simulink model "ES200A_CurrMeas"  (R2013b)
settings: Solver=FixedStepDiscrete  SolverMode=SingleTasking  StartTime=0.0  StopTime=1  FixedStep=0.000125  RelTol=1e-3
values from neighbouring files (symbols this model uses):
  ARCHGLBPRM_2PI_ULS_F32 = DataDict.Constant    [ES200A_CurrMeas_DataDict.m]
  CurrMeasEolGainMax = DataDict.Calibration    [ES200A_CurrMeas_DataDict.m]
  CurrMeasEolGainMin = DataDict.Calibration    [ES200A_CurrMeas_DataDict.m]
  CurrMeasEolGainNrOfSample = DataDict.Calibration    [ES200A_CurrMeas_DataDict.m]
  CurrMeasEolGainNumer = DataDict.Calibration    [ES200A_CurrMeas_DataDict.m]
  CurrMeasEolMaxMotVel = DataDict.Calibration    [ES200A_CurrMeas_DataDict.m]
  CurrMeasEolOffsHiBrdgVltgMin = DataDict.Calibration    [ES200A_CurrMeas_DataDict.m]
  CurrMeasEolOffsHiCmuOffs = DataDict.Calibration    [ES200A_CurrMeas_DataDict.m]
  CurrMeasEolOffsLoCmuOffs = DataDict.Calibration    [ES200A_CurrMeas_DataDict.m]
  CurrMeasEolOffsMax = DataDict.Calibration    [ES200A_CurrMeas_DataDict.m]
  CurrMeasEolOffsMin = DataDict.Calibration    [ES200A_CurrMeas_DataDict.m]
  CurrMeasEolOffsNrOfSample = DataDict.Calibration    [ES200A_CurrMeas_DataDict.m]
  CurrMeasEolTranCntrThd = DataDict.Calibration    [ES200A_CurrMeas_DataDict.m]
  CurrMeasMinRqrdPhaOnTi = DataDict.Calibration    [ES200A_CurrMeas_DataDict.m]
  CurrMeasMotAgCompuDly = DataDict.Calibration    [ES200A_CurrMeas_DataDict.m]
  CurrMeasMotCurrAdcVlyWrmIninMax = DataDict.Calibration    [ES200A_CurrMeas_DataDict.m]
  CurrMeasMotCurrAdcVlyWrmIninMin = DataDict.Calibration    [ES200A_CurrMeas_DataDict.m]
  CurrMeasNtc0x05DFailStep = DataDict.Calibration    [ES200A_CurrMeas_DataDict.m]
  CurrMeasNtc0x05DPassStep = DataDict.Calibration    [ES200A_CurrMeas_DataDict.m]
  CurrMeasNtc0x06DFailStep = DataDict.Calibration    [ES200A_CurrMeas_DataDict.m]
  CurrMeasNtc0x06DPassStep = DataDict.Calibration    [ES200A_CurrMeas_DataDict.m]
  DEGREES30_MOTRAD_F32 = DataDict.Constant    [ES200A_CurrMeas_DataDict.m]
  DIFOFFSRNGCHKMAX_VOLT_F32 = DataDict.Constant    [ES200A_CurrMeas_DataDict.m]
  ELECGLBPRM_IVTRCNT_CNT_U08 = DataDict.ConfigParam    [ES200A_CurrMeas_DataDict.m]
  ELECGLBPRM_STRTUPSTCURRMEASWRMININTESTSTRT_CNT_U08 = DataDict.Constant    [ES200A_CurrMeas_DataDict.m]
  FLTINJ_CURRMEAS_MOTCURRCORRDA = DataDict.Constant    [ES200A_CurrMeas_DataDict.m]
  FLTINJ_CURRMEAS_MOTCURRCORRDD = DataDict.Constant    [ES200A_CurrMeas_DataDict.m]
  FLTINJ_CURRMEAS_TESTOK = DataDict.Constant    [ES200A_CurrMeas_DataDict.m]
  MAXCURRCORRD_AMPR_F32 = DataDict.Constant    [ES200A_CurrMeas_DataDict.m]
  PhaABCMeasdOutOfRng = DataDict.NTC    [ES200A_CurrMeas_DataDict.m]
  PhaDEFMeasOutOfRng = DataDict.NTC    [ES200A_CurrMeas_DataDict.m]
  SysGlbPrmMotPoleCnt = DataDict.ImprtdCal    [ES200A_CurrMeas_DataDict.m]
libraries: simulink x10, FixdToFloat x1
(part 7 of 7)

== stateflow chart ES200A_CurrMeas/CurrMeas/CurrMeasPer2/Chart1 ==
  state PrtclChkENABC = ProtocolChkENABC(MotCtrlMotCurrAdcVlyAAdcFaild,MotCtrlMotCurrAdcVlyBAdcFaild,MotCtrlMotCurrAdcVlyCAdcFaild) [function]
  state PrtclChkENDEF = ProtocolChkENDEF(MotCtrlMotCurrAdcVlyDAdcFaild,MotCtrlMotCurrAdcVlyEAdcFaild,MotCtrlMotCurrAdcVlyFAdcFaild) [function]
  state [MotCurrOffsA,MotCurrOffsB,MotCurrOffsC] = OffsCalcABC(MotCtrlPhaOnTiA,MotCtrlPhaOnTiB,MotCtrlPhaOnTiC,MotCtrlBrdgVltg,MotCurrOffsDeltaA,MotCurrOffsDeltaB,... [function]
    MotCurrOffsDeltaC,CurrMeasEolOffsLoCmuOffs,MotCurrOffsLoAvrgA,MotCurrOffsLoAvrgB,MotCurrOffsLoAvrgC)
  state [MotCurrOffsD,MotCurrOffsE,MotCurrOffsF] = OffsCalcDEF(MotCurrOffsDeltaD,MotCurrOffsDeltaE,MotCurrOffsDeltaF,MotCtrlBrdgVltg,MotCurrOffsLoAvrgD,... [function]
    MotCurrOffsLoAvrgE,MotCurrOffsLoAvrgF,MotCtrlPhaOnTiA,MotCtrlPhaOnTiB,MotCtrlPhaOnTiC,CurrMeasEolOffsLoCmuOffs)
  state MotCtrlCurrMeasMotAgCorrd = CalcMotCurrMotAgCorrd(MotCtrlMotAgElec,MotCtrlMotElecMeclPolarity,MotCtrlMotVelMrf,CurrMeasMotAgCompuDly) [function]
  note: ***Rev 4.5.0 Change****************************
  note: *****Rationale*******************************************
      | MotCtrlPhaOnTi is a percentage of MotCtrlPwmPerd
      | Therefore, MotCtrlPhaOnTi is always less than
      | or equal to MotCtrlPwmPerd
      | **********************************************************
  (default) -> (junction 146)
  (junction 146) -> (junction 14) [order 2]
  (junction 146) -> (junction 104) [order 1] : [((MotCtrlSysSt == 2) || (MotCtrlSysSt == 3)) && (MotCtrlCurrMeasWrmIninTestCmplPrev == 1)]
  (junction 14) -> (junction 254)
  (junction 104) -> (junction 38) [order 2] : {PrtclChkENABC = 0;}
  (junction 104) -> (junction 93) [order 1] : [MotCtrlDiagcStsIvtr1Inactv == 0]
  (junction 93) -> (junction 142) : {PrtclChkENABC = ProtocolChkENABC(MotCtrlMotCurrAdcVlyAAdcFaild, MotCtrlMotCurrAdcVlyBAdcFaild, ...
      | MotCtrlMotCurrAdcVlyCAdcFaild);}
  (junction 142) -> (junction 163) [order 2]
  (junction 163) -> (junction 165) [order 2] : {MotCtrlNtc5DErrCnt = MotCtrlNtc5DErrCntPrev + 1;}
  (junction 163) -> (junction 165) [order 1] : [MotCtrlNtc5DErrCntPrev == 65535]
      | {MotCtrlNtc5DErrCnt = 0;}
  (junction 142) -> (junction 115) [order 1] : [PrtclChkENABC == 1]
      | {[MotCurrOffsA,MotCurrOffsB,MotCurrOffsC] = OffsCalcABC(MotCtrlPhaOnTiA, MotCtrlPhaOnTiB,MotCtrlPhaOnTiC, MotCtrlBrdgVltg, MotCurrOffsDeltaA,...
      | MotCurrOffsDeltaB, MotCurrOffsDeltaC, CurrMeasEolOffsLoCmuOffs, MotCurrOffsLoAvrgA, MotCurrOffsLoAvrgB, MotCurrOffsLoAvrgC);}
  (junction 115) -> (junction 38) [order 2] : {MotCtrlMotCurrRollgCntr1 = 0;}
  (junction 115) -> (junction 38) [order 1] : [MotCtrlMotCurrRollgCntr1 < 255]
      | {MotCtrlMotCurrRollgCntr1 = MotCurrRollgCnt1Prev + 1;}
  (junction 165) -> (junction 38)
  (junction 38) -> (junction 143) [order 2] : {PrtclChkENDEF = 0;}
  (junction 38) -> (junction 75) [order 1] : [MotCtrlDiagcStsIvtr2Inactv == 0 && ELECGLBPRM_IVTRCNT_CNT_U08 == 2]
  (junction 75) -> (junction 19) : {PrtclChkENDEF = ProtocolChkENDEF(MotCtrlMotCurrAdcVlyDAdcFaild,MotCtrlMotCurrAdcVlyEAdcFaild, ...
      | MotCtrlMotCurrAdcVlyFAdcFaild);}
  (junction 19) -> (junction 170) [order 2]
  (junction 170) -> (junction 167) [order 2] : {MotCtrlNtc6DErrCnt = MotCtrlNtc6DErrCntPrev + 1;}
  (junction 19) -> (junction 8) [order 1] : [PrtclChkENDEF == 1]
      | {[MotCurrOffsD,MotCurrOffsE,MotCurrOffsF] = OffsCalcDEF(MotCurrOffsDeltaD, MotCurrOffsDeltaE, MotCurrOffsDeltaF, MotCtrlBrdgVltg,...
      | MotCurrOffsLoAvrgD, MotCurrOffsLoAvrgE, MotCurrOffsLoAvrgF, MotCtrlPhaOnTiA, MotCtrlPhaOnTiB, MotCtrlPhaOnTiC, CurrMeasEolOffsLoCmuOffs);}
  (junction 170) -> (junction 167) [order 1] : [MotCtrlNtc6DErrCntPrev == 65535]
      | {MotCtrlNtc6DErrCnt = 0;}
  (junction 8) -> (junction 143) [order 2] : {MotCtrlMotCurrRollgCntr2 = 0;}
  (junction 8) -> (junction 143) [order 1] : [MotCtrlMotCurrRollgCntr2 < 255]
      | {MotCtrlMotCurrRollgCntr2 = MotCurrRollgCnt2Prev +1;}
  (junction 167) -> (junction 143)
  (junction 143) -> (junction 80)
  (junction 103) -> (junction 159) [order 2]
  (junction 29) -> (junction 96) : {MotCtrlMotCurrCorrdD = (MotCtrlMotCurrAdcVlyD - MotCurrOffsD) * (-MotCurrEolGainD);
      | MotCtrlMotCurrCorrdE = (MotCtrlMotCurrAdcVlyE - MotCurrOffsE) * (-MotCurrEolGainE);
      | MotCtrlMotCurrCorrdF = (MotCtrlMotCurrAdcVlyF - MotCurrOffsF) * (-MotCurrEolGainF);}
  (junction 103) -> (junction 87) [order 1] : [PrtclChkENABC == 1]
  (junction 87) -> (junction 159) : {MotCtrlMotCurrCorrdA = (MotCtrlMotCurrAdcVlyA - MotCurrOffsA) * (-MotCurrEolGainA);
      | MotCtrlMotCurrCorrdB = (MotCtrlMotCurrAdcVlyB - MotCurrOffsB) * (-MotCurrEolGainB);
      | MotCtrlMotCurrCorrdC = (MotCtrlMotCurrAdcVlyC - MotCurrOffsC) * (-MotCurrEolGainC);}
  (junction 80) -> (junction 103) [order 1] : [(MotCtrlPwmPerd - MotCtrlPhaOnTiA) > CurrMeasMinRqrdPhaOnTi && ...
      |  (MotCtrlPwmPerd - MotCtrlPhaOnTiB) > CurrMeasMinRqrdPhaOnTi && ...
      | (MotCtrlPwmPerd - MotCtrlPhaOnTiC) > CurrMeasMinRqrdPhaOnTi]
  (junction 159) -> (junction 29) [order 1] : [PrtclChkENDEF == 1]
  (junction 96) -> (junction 148)
  (junction 159) -> (junction 50) [order 2]
  (junction 80) -> (junction 114) [order 2]
  (junction 84) -> (junction 151) [order 2]
  (junction 101) -> (junction 148) : {MotCtrlMotCurrCorrdE = (MotCtrlMotCurrAdcVlyE - MotCurrOffsE) * (-MotCurrEolGainE);
      | MotCtrlMotCurrCorrdF = (MotCtrlMotCurrAdcVlyF - MotCurrOffsF) * (-MotCurrEolGainF);
      | MotCtrlMotCurrCorrdD = - MotCtrlMotCurrCorrdE - MotCtrlMotCurrCorrdF;}
  (junction 114) -> (junction 84) [order 1] : [(MotCtrlPwmPerd - MotCtrlPhaOnTiA) < CurrMeasMinRqrdPhaOnTi && ...
      |  (MotCtrlPwmPerd - MotCtrlPhaOnTiB) > CurrMeasMinRqrdPhaOnTi && ...
      | (MotCtrlPwmPerd - MotCtrlPhaOnTiC) > CurrMeasMinRqrdPhaOnTi]
  (junction 84) -> (junction 88) [order 1] : [PrtclChkENABC == 1]
  (junction 88) -> (junction 151) : {MotCtrlMotCurrCorrdB = (MotCtrlMotCurrAdcVlyB - MotCurrOffsB) * (-MotCurrEolGainB);
      | MotCtrlMotCurrCorrdC = (MotCtrlMotCurrAdcVlyC - MotCurrOffsC) * (-MotCurrEolGainC);
      | MotCtrlMotCurrCorrdA = - MotCtrlMotCurrCorrdB - MotCtrlMotCurrCorrdC;}
  (junction 151) -> (junction 101) [order 1] : [PrtclChkENDEF == 1]
  (junction 148) -> (junction 77)
  (junction 151) -> (junction 50) [order 2]
  (junction 114) -> (junction 26) [order 2]
  (junction 147) -> (junction 48) [order 2]
  (junction 79) -> (junction 77) : {MotCtrlMotCurrCorrdD = (MotCtrlMotCurrAdcVlyD - MotCurrOffsD) * (-MotCurrEolGainD);
      | MotCtrlMotCurrCorrdF = (MotCtrlMotCurrAdcVlyF - MotCurrOffsF) * (-MotCurrEolGainF);
      | MotCtrlMotCurrCorrdE = - MotCtrlMotCurrCorrdD - MotCtrlMotCurrCorrdF;}
  (junction 26) -> (junction 147) [order 1] : [(MotCtrlPwmPerd - MotCtrlPhaOnTiA) > CurrMeasMinRqrdPhaOnTi && ...
      |  (MotCtrlPwmPerd - MotCtrlPhaOnTiB) < CurrMeasMinRqrdPhaOnTi && ...
      | (MotCtrlPwmPerd - MotCtrlPhaOnTiC) > CurrMeasMinRqrdPhaOnTi]
  (junction 147) -> (junction 32) [order 1] : [PrtclChkENABC == 1]
  (junction 32) -> (junction 48) : {MotCtrlMotCurrCorrdA = (MotCtrlMotCurrAdcVlyA - MotCurrOffsA) * (-MotCurrEolGainA);
      | MotCtrlMotCurrCorrdC = (MotCtrlMotCurrAdcVlyC - MotCurrOffsC) * (-MotCurrEolGainC);
      | MotCtrlMotCurrCorrdB = - MotCtrlMotCurrCorrdA - MotCtrlMotCurrCorrdC;}
  (junction 48) -> (junction 79) [order 1] : [PrtclChkENDEF == 1]
  (junction 77) -> (junction 30)
  (junction 48) -> (junction 50) [order 2]
  (junction 26) -> (junction 113) [order 2]
  (junction 122) -> (junction 76) [order 2]
  (junction 36) -> (junction 30) : {MotCtrlMotCurrCorrdD = (MotCtrlMotCurrAdcVlyD - MotCurrOffsD) * (-MotCurrEolGainD);
      | MotCtrlMotCurrCorrdE = (MotCtrlMotCurrAdcVlyE - MotCurrOffsE) * (-MotCurrEolGainE);
      | MotCtrlMotCurrCorrdF = - MotCtrlMotCurrCorrdD - MotCtrlMotCurrCorrdD;}
  (junction 122) -> (junction 117) [order 1] : [PrtclChkENABC == 1]
  (junction 113) -> (junction 122) [order 1] : [(MotCtrlPwmPerd - MotCtrlPhaOnTiA) > CurrMeasMinRqrdPhaOnTi && ...
      |  (MotCtrlPwmPerd - MotCtrlPhaOnTiB) > CurrMeasMinRqrdPhaOnTi && ...
      | (MotCtrlPwmPerd - MotCtrlPhaOnTiC) < CurrMeasMinRqrdPhaOnTi]
  (junction 117) -> (junction 76) : {MotCtrlMotCurrCorrdA = (MotCtrlMotCurrAdcVlyA - MotCurrOffsA) * (-MotCurrEolGainA);
      | MotCtrlMotCurrCorrdB = (MotCtrlMotCurrAdcVlyB - MotCurrOffsB) * (-MotCurrEolGainB);
      | MotCtrlMotCurrCorrdC = - MotCtrlMotCurrCorrdA - MotCtrlMotCurrCorrdB;}
  (junction 76) -> (junction 36) [order 1] : [PrtclChkENDEF == 1]
  (junction 30) -> (junction 119)
  (junction 76) -> (junction 50) [order 2]
  (junction 113) -> (junction 95) [order 2]
  (junction 95) -> (junction 50) : {CurrMeasPhaOnTiErrCnt = CurrMeasPhaOnTiErrCntPrev +1;}
  (junction 119) -> (junction 50)
  (junction 50) -> (junction 25) : {
      | MotCtrlCurrMeasMotAgCorrd = CalcMotCurrMotAgCorrd(MotCtrlMotAgElec, MotCtrlMotElecMeclPolarity, MotCtrlMotVelMrf, CurrMeasMotAgCompuDly);
      | }
  (junction 254) -> (junction 25)
  data: MotCtrlMotCurrAdcVlyAAdcFaild function_input; MotCtrlMotCurrAdcVlyBAdcFaild function_input; MotCtrlMotCurrAdcVlyCAdcFaild function_input; PrtclChkENABC function_output; PrtclChkENDEF function_output; MotCtrlMotCurrAdcVlyDAdcFaild function_input; MotCtrlMotCurrAdcVlyEAdcFaild function_input; MotCtrlMotCurrAdcVlyFAdcFaild function_input; MotCtrlPhaOnTiA function_input; MotCtrlPhaOnTiB function_input; MotCtrlPhaOnTiC function_input; MotCtrlBrdgVltg function_input; MotCurrOffsDeltaA function_input; MotCurrOffsDeltaB function_input; MotCurrOffsDeltaC function_input; CurrMeasEolOffsLoCmuOffs function_input; MotCurrOffsLoAvrgA function_input; MotCurrOffsLoAvrgB function_input; MotCurrOffsLoAvrgC function_input; MotCurrOffsA function_output; MotCurrOffsB function_output; MotCurrOffsC function_output; MotCurrOffsDeltaD function_input; MotCurrOffsDeltaE function_input; MotCurrOffsDeltaF function_input; MotCtrlBrdgVltg function_input; MotCurrOffsLoAvrgD function_input; MotCurrOffsLoAvrgE function_input; MotCurrOffsLoAvrgF function_input; MotCtrlPhaOnTiA function_input; MotCtrlPhaOnTiB function_input; MotCtrlPhaOnTiC function_input; CurrMeasEolOffsLoCmuOffs function_input; MotCurrOffsD function_output; MotCurrOffsE function_output; MotCurrOffsF function_output; MotCtrlMotAgElec function_input; MotCtrlMotElecMeclPolarity function_input; MotCtrlMotVelMrf function_input; CurrMeasMotAgCompuDly function_input; MotCtrlCurrMeasMotAgCorrd function_output; MotCtrlMotCurrAdcVlyA input; MotCtrlMotCurrAdcVlyB input; MotCtrlMotCurrAdcVlyC input; MotCtrlMotCurrAdcVlyD input; MotCtrlMotCurrAdcVlyE input; MotCtrlMotCurrAdcVlyF input; MotCtrlMotCurrAdcVlyAAdcFaild input; MotCtrlMotCurrAdcVlyBAdcFaild input; MotCtrlMotCurrAdcVlyCAdcFaild input; MotCtrlMotCurrAdcVlyDAdcFaild input; MotCtrlMotCurrAdcVlyEAdcFaild input; MotCtrlMotCurrAdcVlyFAdcFaild input; CurrMeasEolOffsLoCmuOffs input; CurrMeasMinRqrdPhaOnTi input; CurrMeasMotAgCompuDly input; MotCtrlBrdgVltg input; MotCtrlDiagcStsIvtr1Inactv input; MotCtrlDiagcStsIvtr2Inactv input; MotCtrlMotAgElec input; MotCtrlMotElecMeclPolarity input; MotCtrlMotVelMrf input; MotCtrlPhaOnTiA input; MotCtrlPhaOnTiB input; MotCtrlPhaOnTiC input; MotCtrlPwmPerd input; MotCtrlSysSt input; MotCurrEolGainA input; MotCurrEolGainB input; MotCurrEolGainC input; MotCurrEolGainD input; MotCurrEolGainE input; MotCurrEolGainF input; MotCurrOffsDeltaA input; MotCurrOffsDeltaB input; MotCurrOffsDeltaC input; MotCurrOffsDeltaD input; MotCurrOffsDeltaE input; MotCurrOffsDeltaF input; MotCurrOffsLoAvrgA input; MotCurrOffsLoAvrgB input; MotCurrOffsLoAvrgC input; MotCurrOffsLoAvrgD input; MotCurrOffsLoAvrgE input; MotCurrOffsLoAvrgF input; ELECGLBPRM_IVTRCNT_CNT_U08 input; MotCtrlCurrMeasWrmIninTestCmplPrev input boolean; MotCtrlNtc5DErrCntPrev input uint16; MotCtrlNtc6DErrCntPrev input uint16; MotCurrRollgCnt1Prev input; MotCurrRollgCnt2Prev input; MotCtrlCurrMeasMotAgCorrd output double; MotCtrlMotCurrCorrdA output single; MotCtrlMotCurrCorrdB output single; MotCtrlMotCurrCorrdC output single; MotCtrlMotCurrCorrdD output single; MotCtrlMotCurrCorrdE output single; MotCtrlMotCurrCorrdF output single; MotCtrlNtc5DErrCnt output uint16; MotCtrlNtc6DErrCnt output uint16; MotCtrlMotCurrRollgCntr1 output uint8; MotCtrlMotCurrRollgCntr2 output uint8; MotCurrOffsA local double; MotCurrOffsB local double; MotCurrOffsC local double; MotCurrOffsD local double; MotCurrOffsE local double; MotCurrOffsF local double; CurrMeasPhaOnTiErrCntPrev input; CurrMeasPhaOnTiErrCnt output uint16; PrtclChkENABC local double; PrtclChkENDEF local double

== stateflow chart ES200A_CurrMeas/CurrMeas/CurrMeasPer3/Chart1/SetNtc5DSts/SetNtcSts/ISO Fault Debounce Design ==
  note: NTCSTS_PASSD           (0)
      | NTCSTS_FAILD             (1)
      | NTCSTS_PREPASSD   (2)
      | NTCSTS_PREFAILD     (3)
      |
      | SIGQLFR_NORES        (0)
      | SIGQLFR_PASSD         (1)
      | SIGQLFR_FAILD           (2)
  note: Pass Loop
  note: Fail Loop
  note: 
  note: Moved condition Action {ErrAcc = 0;
      | Qualifier =0;
      | } from 2nd Transition action to first trnasition action as there is no condition action in first transition action
      | Also changed SvcClr to 1
  (default) -> (junction 89)
  (junction 89) -> (junction 95) [order 1] : [NtcSts ==3]
  (junction 89) -> (junction 93) [order 2] : [NtcSts ==2]
  (junction 89) -> (junction 141) [order 3] : [NtcSts ==1]
      | { ErrAcc = 32767;
      | Qualifier =2;
      |  }
  (junction 89) -> (junction 141) [order 4] : [NtcSts ==0]
      | { ErrAcc = -32768;
      | Qualifier=1;
      | }
  (junction 95) -> (junction 103) [order 2]
  (junction 95) -> (junction 111) [order 1] : [ErrAcc <=0]
      | {ErrAcc = DebStep;}
  (junction 93) -> (junction 123) [order 2] : {
      | ErrAcc = ErrAcc - DebStep;
      | }
  (junction 93) -> (junction 123) [order 1] : [(ErrAcc - DebStep) <= -32768]
      | { ErrAcc = -32768;
      | Qualifier=1;
      | }
  (junction 103) -> (junction 111) [order 1] : [(ErrAcc + DebStep) <32767]
      | {ErrAcc = ErrAcc + DebStep;}
  (junction 103) -> (junction 111) [order 2] : {ErrAcc = 32767;
      | Qualifier =2;}
  (junction 123) -> (junction 141)
  (junction 111) -> (junction 141)
  (junction 141) -> (junction 159) [order 2]
  (junction 141) -> (junction 159) [order 1] : [SvcClr ==1]
      | {ErrAcc = 0;
      | Qualifier =0;
      | }
  data: NtcSts input uint8; Qualifier output uint8; DebStep input int32; ErrAcc local single; SvcClr input

== stateflow chart ES200A_CurrMeas/CurrMeas/CurrMeasPer3/Chart1 ==
  note: /*    if [CurrMeasMotCurrAdcVlyWrmIninMin < MotCtrlMotCurrAdcVlyA < CurrMeasMotCurrAdcVlyWrmIninMax &&...
      |           CurrMeasMotCurrAdcVlyWrmIninMin < MotCtrlMotCurrAdcVlyB < CurrMeasMotCurrAdcVlyWrmIninMax &&...
      |           CurrMeasMotCurrAdcVlyWrmIninMin < MotCtrlMotCurrAdcVlyC < CurrMeasMotCurrAdcVlyWrmIninMax]
      |         {
      |           RangeCheckWIABC == 1;
      |          } */
  state MotCurrNtcSet1 = SetNtc5DSts(NTCNr,ParamBit,NTCSts,NTCDebStep) [function]
  state RangeCheckWIABC = RangeChkWIABC(MotCtrlMotCurrAdcVlyA,MotCtrlMotCurrAdcVlyB,MotCtrlMotCurrAdcVlyC) [function]
  note: Note:
      | Function call to be used in the code is "SetNtcSts" instead of "SetNtc5DSts"
      | "SetNtc5DSts" is used only to simulate the diag manager.
  state RangeCheckWIDEF = RangeChkWIDEF(MotCtrlMotCurrAdcVlyD,MotCtrlMotCurrAdcVlyE,MotCtrlMotCurrAdcVlyF) [function]
  state MotCurrNtcSet2 = SetNtc6DSts(NTCNr,ParamBit,NTCSts,NTCDebStep) [function]
  note: Note:
      | Function call to be used in the code is "SetNtcSts" instead of "SetNtc6DSts"
      | "SetNtc6DSts" is used only to simulate the diag manager.
  state NtcQlfr = GetNtc5DQlfrSts(NtcNr) [function]
  note: Note:
      | Function call to be used in the code is "GetNtcQlfrSts"
      | instead of "GetNtc5DQlfrSts"
      | "GetNtc5DQlfrSts" is used only to simulate the diag manager.
  note: Note:
      | Function call to be used in the code is "GetNtcQlfrSts"
      | instead of "GetNtc5DQlfrSts"
      | "GetNtc5DQlfrSts" is used only to simulate the diag manager.
  note: /*IvtrCnt = 1 */
  state NtcQlfr = GetNtc6DQlfrSts(NtcNr) [function]
  note: Note:
      | Function call to be used in the code is "GetNtcQlfrSts"
      | instead of "GetNtc6DQlfrSts"
      | "GetNtc6DQlfrSts" is used only to simulate the diag manager.
  note: Note:
      | Function call to be used in the code is "GetNtcQlfrSts"
      | instead of "GetNtc6DQlfrSts"
      | "GetNtc6DQlfrSts" is used only to simulate the diag manager.
  (default) -> (junction 443) : {CurrMeasWrmIninTestCmpl = CurrMeasWrmIninTestCmplPrev;}
  (junction 443) -> (junction 169) [order 2]
  (junction 443) -> (junction 447) [order 1] : [((SysSt == 2) || (SysSt == 3)) && (CurrMeasWrmIninTestCmpl == 1)]
  (junction 169) -> (junction 170) [order 2] : {CurrMeasWrmIninTestCmpl = 0;}
  (junction 447) -> (junction 520) [order 1] : /* Ntc5DErrCnt NOT incremented - PassStep*/
      | [Ntc5DErrCnt == Ntc5DErrCnt2MsPrev]
      | {MotCurrNtcSet1 = SetNtc5DSts(PhaABCMeasdOutOfRng, 0, 2, CurrMeasNtc0x05DPassStep);}
  (junction 447) -> (junction 508) [order 2] : /* Ntc5DErrCnt incremented - FailStep*/
  (junction 169) -> (junction 168) [order 1] : [(SysSt == 3) && (StrtUpSt == ELECGLBPRM_STRTUPSTCURRMEASWRMININTESTSTRT_CNT_U08) ]
  (junction 170) -> (junction 163) : {MotCurrQlfr1 = GetNtc5DQlfrSts(PhaABCMeasdOutOfRng);
      | MotCurrQlfr2 = GetNtc6DQlfrSts(PhaDEFMeasOutOfRng);}
  (junction 168) -> (junction 425) [order 2]
  (junction 425) -> (junction 428)
  (junction 168) -> (junction 217) [order 1] : [DiagcStsIvtr1Inactv == 0]
  (junction 508) -> (junction 510) [order 2] : {ParamABC = 3;}    /* Failed at Warm Init*/
  (junction 508) -> (junction 509) [order 1] : [SysSt == 2]
      | {ParamABC = 2;}
  (junction 217) -> (junction 222) : {RangeCheckWIABC = RangeChkWIABC(MotCtrlMotCurrAdcVlyA, MotCtrlMotCurrAdcVlyB, ...
      | MotCtrlMotCurrAdcVlyC);}
  (junction 510) -> (junction 513)
  (junction 509) -> (junction 513)
  (junction 222) -> (junction 435) [order 2]
  (junction 513) -> (junction 520) : {MotCurrNtcSet1 = SetNtc5DSts(PhaABCMeasdOutOfRng, ParamABC, 3, CurrMeasNtc0x05DFailStep);}
  (junction 222) -> (junction 427) [order 1] : [RangeCheckWIABC == 1]
      | {MotCurrNtcSet1 = SetNtc5DSts(PhaABCMeasdOutOfRng, 0, 2, CurrMeasNtc0x05DPassStep);}
  (junction 435) -> (junction 436) : {MotCurrNtcSet1 = SetNtc5DSts(PhaABCMeasdOutOfRng, 1, 3, CurrMeasNtc0x05DFailStep);}
  (junction 520) -> (junction 540)
  (junction 428) -> (junction 427)
  (junction 436) -> (junction 427)
  (junction 427) -> (junction 215)
  (junction 215) -> (junction 426) [order 2]
  (junction 540) -> (junction 549) [order 1] : /* Ntc5DErrCnt NOT incremented - PassStep*/
      | [Ntc6DErrCnt == Ntc6DErrCnt2MsPrev]
      | {MotCurrNtcSet1 = SetNtc6DSts(PhaDEFMeasOutOfRng, 0, 2, CurrMeasNtc0x06DPassStep);}
  (junction 426) -> (junction 432)
  (junction 215) -> (junction 228) [order 1] : [DiagcStsIvtr2Inactv == 0 && ELECGLBPRM_IVTRCNT_CNT_U08 == 2]
  (junction 540) -> (junction 551) [order 2] : /* Ntc6DErrCnt incremented */
  (junction 228) -> (junction 221) : {RangeCheckWIDEF = RangeChkWIDEF(MotCtrlMotCurrAdcVlyD, MotCtrlMotCurrAdcVlyE, ...
      | MotCtrlMotCurrAdcVlyF );}
  (junction 551) -> (junction 545) [order 2] : {ParamDEF = 3;}   /* Failed at Warm Init*/
  (junction 551) -> (junction 554) [order 1] : [SysSt == 2]
      | {ParamDEF = 2;}
  (junction 545) -> (junction 555)
  (junction 554) -> (junction 555)
  (junction 221) -> (junction 439) [order 2]
  (junction 221) -> (junction 231) [order 1] : [RangeCheckWIDEF == 1]
      | {MotCurrNtcSet2 = SetNtc6DSts(PhaDEFMeasOutOfRng, 0, 2, CurrMeasNtc0x06DPassStep);}
  (junction 439) -> (junction 440) : {MotCurrNtcSet2 = SetNtc6DSts(PhaDEFMeasOutOfRng, 1, 3, CurrMeasNtc0x06DFailStep);}
  (junction 555) -> (junction 549) : {MotCurrNtcSet1 = SetNtc6DSts(PhaDEFMeasOutOfRng, ParamDEF, 3, CurrMeasNtc0x06DFailStep);}
  (junction 549) -> (junction 493)
  (junction 432) -> (junction 231)
  (junction 440) -> (junction 231)
  (junction 231) -> (junction 164) : {MotCurrQlfr1 = GetNtc5DQlfrSts(PhaABCMeasdOutOfRng);
      | MotCurrQlfr2 = GetNtc6DQlfrSts(PhaDEFMeasOutOfRng);}
  (junction 164) -> (junction 162) [order 2] : /* [(DiagcStsIvtr1Inactv == 0 || DiagcStsIvtr2Inactv == 0)] */
  (junction 164) -> (junction 160) [order 1] : [DiagcStsIvtr1Inactv == 0 &&...
      | DiagcStsIvtr2Inactv == 0 &&...
      | ELECGLBPRM_IVTRCNT_CNT_U08 == 2]
  (junction 493) -> (junction 455) : {MotCurrQlfr1 = GetNtc5DQlfrSts(PhaABCMeasdOutOfRng);
      | MotCurrQlfr2 = GetNtc6DQlfrSts(PhaDEFMeasOutOfRng);}
  (junction 162) -> (junction 159) [order 1] : [MotCurrQlfr1 > 0 || MotCurrQlfr2 > 0]
      | {CurrMeasWrmIninTestCmpl = 1;}
  (junction 160) -> (junction 159) [order 1] : [MotCurrQlfr1 > 0 && MotCurrQlfr2 > 0]
      | {CurrMeasWrmIninTestCmpl = 1;}
  (junction 160) -> (junction 421) [order 2]
  (junction 162) -> (junction 422) [order 2]
  (junction 159) -> (junction 158)
  (junction 455) -> (junction 421) : {Ntc5DErrCnt2Ms = Ntc5DErrCnt;
      |  Ntc6DErrCnt2Ms = Ntc6DErrCnt;}
  (junction 421) -> (junction 158)
  (junction 422) -> (junction 158)
  (junction 163) -> (junction 422)
  data: NTCNr function_input; ParamBit function_input; NTCSts function_input; NTCDebStep function_input; MotCurrNtcSet1 function_output; RangeCheckWIABC function_output; MotCtrlMotCurrAdcVlyA function_input; MotCtrlMotCurrAdcVlyB function_input; MotCtrlMotCurrAdcVlyC function_input; RangeCheckWIDEF function_output; MotCtrlMotCurrAdcVlyD function_input; MotCtrlMotCurrAdcVlyE function_input; MotCtrlMotCurrAdcVlyF function_input; NTCNr function_input; ParamBit function_input; NTCSts function_input; NTCDebStep function_input; MotCurrNtcSet2 function_output; NtcNr function_input; NtcQlfr function_output; NtcNr function_input; NtcQlfr function_output; CurrMeasNtc0x05DFailStep input; CurrMeasNtc0x05DPassStep input; CurrMeasNtc0x06DFailStep input; CurrMeasNtc0x06DPassStep input; DiagcStsIvtr1Inactv input; DiagcStsIvtr2Inactv input; Ntc5DErrCnt input; Ntc6DErrCnt input uint16; StrtUpSt input; SysSt input; MotCurrNtcSet1 local double; MotCurrNtcSet2 local double; MotCurrQlfr1 output double; MotCurrQlfr2 output double; RangeCheckWIABC local double; RangeCheckWIDEF local double; ELECGLBPRM_IVTRCNT_CNT_U08 input; PhaABCMeasdOutOfRng input; PhaDEFMeasOutOfRng input; ELECGLBPRM_STRTUPSTCURRMEASWRMININTESTSTRT_CNT_U08 input uint8; CurrMeasWrmIninTestCmplPrev input boolean; Ntc5DErrCnt2Ms output uint16; Ntc6DErrCnt2Ms output uint16; CurrMeasWrmIninTestCmpl output boolean; ParamABC local double; ParamDEF local double; MotCtrlMotCurrAdcVlyA input; MotCtrlMotCurrAdcVlyB input; MotCtrlMotCurrAdcVlyC input; MotCtrlMotCurrAdcVlyD input; MotCtrlMotCurrAdcVlyE input; MotCtrlMotCurrAdcVlyF input; Ntc5DErrCnt2MsPrev input uint16; Ntc6DErrCnt2MsPrev input uint16

== stateflow chart ES200A_CurrMeas/CurrMeas/CurrMeasPer1/Gain Calibration/GainStateMachine ==
  note: EolGainOutOfRng = NTCNR_0X1ED
      | Parameters:
      |     1 = 0000 0001 = Phase A, B, C EOL Calculated Gains are Out Of Range
      |     2 = 0000 0010 = Phase D, E, F EOL Calculated Gains are Out Of Range
      |     3 = 0000 0011 = Phase A, B, C, D, E, F EOL Calculated Gains are Out Of Range
      |     4 = 0000 0100 = VehSpd, VehSpdVld condition not met
      |     8 = 0000 1000 = MotVelMrf condition not met
      |   16 = 0001 0000 = DiagcStsIvtr1Inactv and DiagcStsIvtr1Inactv both TRUE
  note: EolGainSts
      |
      | 0 = Not Started
      | 1 = Started/In Process
      | 2 = Successful
      | 4  = Phase A, B, C EOL Calculated Gains are Out Of Range
      | 8  = Phase D, E, F EOL Calculated Gains are Out Of Range
      | 12 = Phase A, B, C, D, E, F EOL Calculated Gains are Out Of Range
      | 16  = VehSpd, VehSpdVld, condition not met
      | 32  = MotVelMrf condition not met
      | 64 = DiagcStsIvtr1Inactv and DiagcStsIvtr1Inactv both TRUE
  note: ***Rev 4.5.0 Change****************************
      | Replace divisor CurrMeasEolGainNrOfSample
      | with CurrMeasEolAvrgCntr.
      | No functional impact
      | ****************************************************
  note: ***Rev 4.5.0 Change****************************
      | Replace divisor CurrMeasEolGainNrOfSample
      | with CurrMeasEolAvrgCntr.
      | No functional impact
      | ****************************************************
  note: ***Rev 4.5.0 Change****************************
      | Replace divisor CurrMeasEolGainNrOfSample
      | with CurrMeasEolAvrgCntr.
      | No functional impact
      | ****************************************************
  note: Moved transition condition from connective junction 660 to connective junction 661,
      | Transition #620 ([GainRngChkABC == 1 && GainRngChkDEF == 1]
      | {CurrMeasMotCurrEolCalSt = 0;
      | CurrMeasEolAvrgCntr = 0;
      | CurrMeasEolTranCntr = 0;})
  note: EolGainSts
      | 0 = Not Started
      | 1 = Started/In Process
      | 2 = Successful
      | 3 = Not successful
  note: EolGainSts
      |
      | 0 = Not Started
      | 1 = Started/In Process
      | 2 = Successful
      | 4  = Phase A, B, C EOL Calculated Gains are Out Of Range
      | 8  = Phase D, E, F EOL Calculated Gains are Out Of Range
      | 12 = Phase A, B, C, D, E, F EOL Calculated Gains are Out Of Range
      | 16  = VehSpd, VehSpdVld, condition not met
      | 32  = MotVelMrf condition not met
      | 64 = DiagcStsIvtr1Inactv and DiagcStsIvtr1Inactv both TRUE
  state MotCurrNtcSet = SetNtcSts(NTCNr,ParamBit,NTCSts,NTCDebStep) [function]
  note: EolGainOutOfRng = NTCNR_0X1ED
      | Parameters:
      |     1 = 0000 0001 = Phase A, B, C EOL Calculated Gains are Out Of Range
      |     2 = 0000 0010 = Phase D, E, F EOL Calculated Gains are Out Of Range
      |     3 = 0000 0011 = Phase A, B, C, D, E, F EOL Calculated Gains are Out Of Range
      |     4 = 0000 0100 = VehSpd, VehSpdVld condition not met
      |     8 = 0000 1000 = MotVelMrf condition not met
      |   16 = 0001 0000 = DiagcStsIvtr1Inactv and DiagcStsIvtr1Inactv both TRUE
  state WrNvm [function]
  (default) -> (junction 150) : {EolGainSts = EolGainStsPrev;}
  (junction 150) -> (junction 110) [order 2] : {EolGainSts = EolGainStsPrev;}
  (junction 150) -> (junction 78) [order 1] : [EolGainSts == 1 && MotCurrEolOffsProcFlg == 1]
  (junction 78) -> (junction 307) [order 1] : [(VehSpd <= ARCHGLBPRM_FLOATZEROTHD_ULS_F32)...
      |  && (VehSpdVld == 1)]
  (junction 307) -> (junction 79) [order 1] : [(abs(MotVelMrf) <= CurrMeasEolMaxMotVel)]
  (junction 79) -> (junction 76) [order 2]
  (junction 76) -> (junction 105) [order 2]
  (junction 105) -> (junction 133) [order 2]
  (junction 133) -> (junction 136) [order 2]
  (junction 78) -> (junction 110) [order 2] : {CurrMeasMotCurrEolCalSt = MotCurrEolCalSt2.MCECS_CMDSAFEST;
      | MotCurrNtcSet = SetNtcSts(EolGainOutOfRng, 4, 1, 0);
      | EolGainSts = 16;}
  (junction 307) -> (junction 309) [order 2] : {CurrMeasMotCurrEolCalSt = MotCurrEolCalSt2.MCECS_CMDSAFEST;
      | MotCurrNtcSet = SetNtcSts(EolGainOutOfRng, 4, 1, 0);
      | EolGainSts = 32;}
  (junction 79) -> (junction 95) [order 1] : [(CurrMeasMotCurrEolCalStPrev == MotCurrEolCalSt2.MCECS_OFFSCMDEND) ||...
      |  (CurrMeasMotCurrEolCalStPrev == MotCurrEolCalSt2.MCECS_GAINCMDAD)]
      | {CurrMeasMotCurrEolCalSt = MotCurrEolCalSt2.MCECS_GAINCMDAD;}
  (junction 76) -> (junction 88) [order 1] : [CurrMeasMotCurrEolCalStPrev == MotCurrEolCalSt2.MCECS_GAINCMDBE]
  (junction 105) -> (junction 96) [order 1] : [CurrMeasMotCurrEolCalStPrev == MotCurrEolCalSt2.MCECS_GAINCMDCF]
  (junction 133) -> (junction 264) [order 1] : [CurrMeasMotCurrEolCalStPrev == MotCurrEolCalSt2.MCECS_CMDSAFEST]
  (junction 136) -> (junction 131)
  (junction 264) -> (junction 257) [order 2] : {GainRngChkABC = 1;}
  (junction 264) -> (junction 124) [order 1] : [DiagcStsIvtr1Inactv == 0]
  (junction 95) -> (junction 91) [order 2] : {CurrMeasEolTranCntr = CurrMeasEolTranCntrPrev + 1;}
  (junction 96) -> (junction 98) [order 2] : {CurrMeasEolTranCntr = CurrMeasEolTranCntrPrev + 1;}
  (junction 88) -> (junction 104) [order 2] : {CurrMeasEolTranCntr = CurrMeasEolTranCntrPrev + 1;}
  (junction 95) -> (junction 108) [order 1] : [CurrMeasEolTranCntr == CurrMeasEolTranCntrThd]
      |
      | {CurrMeasTmpMotCurrAdcVlySum1 = CurrMeasTmpMotCurrAdcVlySum1Prev + MotCurrAdcVlyA;
      | CurrMeasTmpMotCurrAdcVlySum2 = CurrMeasTmpMotCurrAdcVlySum2Prev + MotCurrAdcVlyD;
      | CurrMeasEolAvrgCntr = CurrMeasEolAvrgCntrPrev + 1;}
  (junction 88) -> (junction 92) [order 1] : [CurrMeasEolTranCntr == CurrMeasEolTranCntrThd]
      |
      | {CurrMeasTmpMotCurrAdcVlySum1 = CurrMeasTmpMotCurrAdcVlySum1Prev + MotCurrAdcVlyB;
      | CurrMeasTmpMotCurrAdcVlySum2 = CurrMeasTmpMotCurrAdcVlySum2Prev + MotCurrAdcVlyE;
      | CurrMeasEolAvrgCntr = CurrMeasEolAvrgCntrPrev + 1;}
  (junction 96) -> (junction 114) [order 1] : [CurrMeasEolTranCntr == CurrMeasEolTranCntrThd]
      |
      | {CurrMeasTmpMotCurrAdcVlySum1 = CurrMeasTmpMotCurrAdcVlySum1Prev + MotCurrAdcVlyC;
      | CurrMeasTmpMotCurrAdcVlySum2 = CurrMeasTmpMotCurrAdcVlySum2Prev + MotCurrAdcVlyF;
      | CurrMeasEolAvrgCntr = CurrMeasEolAvrgCntrPrev + 1;}
  (junction 124) -> (junction 277) [order 2]
  (junction 277) -> (junction 290) : {GainFltParam = 1;
      | GainRngChkABC = 0;}
  (junction 124) -> (junction 257) [order 1] : [(CurrMeasMotCurrEolGainA >= CurrMeasEolGainMin) &&...
      | (CurrMeasMotCurrEolGainA <= CurrMeasEolGainMax) &&...
      | (CurrMeasMotCurrEolGainB >= CurrMeasEolGainMin) &&...
      | (CurrMeasMotCurrEolGainB <= CurrMeasEolGainMax) &&...
      | (CurrMeasMotCurrEolGainC >= CurrMeasEolGainMin) &&...
      | (CurrMeasMotCurrEolGainC <= CurrMeasEolGainMax)]
      |
      | {GainRngChkABC = 1;}
  (junction 290) -> (junction 257)
  (junction 257) -> (junction 120) [order 2] : {GainRngChkDEF = 1;}
  (junction 257) -> (junction 251) [order 1] : [DiagcStsIvtr2Inactv == 0 && ELECGLBPRM_IVTRCNT_CNT_U08 == 2]
  (junction 108) -> (junction 91) [order 2]
  (junction 92) -> (junction 104) [order 2]
  (junction 114) -> (junction 98) [order 2]
  (junction 108) -> (junction 235) [order 1] : [CurrMeasEolAvrgCntr  == CurrMeasEolGainNrOfSample]
      |
      | {MotCurrAvrgA = CurrMeasTmpMotCurrAdcVlySum1 / CurrMeasEolAvrgCntr;
      | MotCurrAvrgD = CurrMeasTmpMotCurrAdcVlySum2 / CurrMeasEolAvrgCntr;}
  (junction 92) -> (junction 238) [order 1] : [CurrMeasEolAvrgCntr  == CurrMeasEolGainNrOfSample]
      |
      | {MotCurrAvrgB = CurrMeasTmpMotCurrAdcVlySum1 / CurrMeasEolAvrgCntr;
      | MotCurrAvrgE = CurrMeasTmpMotCurrAdcVlySum2 / CurrMeasEolAvrgCntr;}
  (junction 114) -> (junction 241) [order 1] : [CurrMeasEolAvrgCntr  == CurrMeasEolGainNrOfSample]
      |
      | {MotCurrAvrgC = CurrMeasTmpMotCurrAdcVlySum1 / CurrMeasEolAvrgCntr;
      | MotCurrAvrgF = CurrMeasTmpMotCurrAdcVlySum2 / CurrMeasEolAvrgCntr;}
  (junction 251) -> (junction 280) [order 2]
  (junction 280) -> (junction 292) : {GainFltParam = GainFltParam + 2;
      | GainRngChkDEF = 0;}
  (junction 251) -> (junction 120) [order 1] : [(CurrMeasMotCurrEolGainD >= CurrMeasEolGainMin) &&...
      | (CurrMeasMotCurrEolGainD <= CurrMeasEolGainMax) &&...
      | (CurrMeasMotCurrEolGainE >= CurrMeasEolGainMin) &&...
      | (CurrMeasMotCurrEolGainE <= CurrMeasEolGainMax) &&...
      | (CurrMeasMotCurrEolGainF >= CurrMeasEolGainMin) &&...
      | (CurrMeasMotCurrEolGainF <= CurrMeasEolGainMax)]
      |
      | {GainRngChkDEF = 1;}
  (junction 292) -> (junction 120)
  (junction 235) -> (junction 91) [order 2] : {CurrMeasEolAvrgCntr = 0;
      | CurrMeasTmpMotCurrAdcVlySum1 = 0;
      | CurrMeasTmpMotCurrAdcVlySum2 = 0;}
  (junction 238) -> (junction 104) [order 2] : {CurrMeasEolAvrgCntr = 0;
      | CurrMeasTmpMotCurrAdcVlySum1 = 0;
      | CurrMeasTmpMotCurrAdcVlySum2 = 0;}
  (junction 241) -> (junction 98) [order 2] : {CurrMeasEolAvrgCntr = 0;
      | CurrMeasTmpMotCurrAdcVlySum1 = 0;
      | CurrMeasTmpMotCurrAdcVlySum2 = 0;}
  (junction 235) -> (junction 91) [order 1] : [abs(MotCurrAvrgA - MotCurrOffsZeroAvrgA) > ARCHGLBPRM_FLOATZEROTHD_ULS_F32 ...
      | && abs(MotCurrAvrgD - MotCurrOffsZeroAvrgD) > ARCHGLBPRM_FLOATZEROTHD_ULS_F32]
      |
      | {CurrMeasMotCurrEolGainA = CurrMeasEolGainNumer / abs(MotCurrAvrgA - MotCurrOffsZeroAvrgA);
      | CurrMeasMotCurrEolGainD = CurrMeasEolGainNumer / abs(MotCurrAvrgD - MotCurrOffsZeroAvrgD);
      |
      | CurrMeasMotCurrEolCalSt = MotCurrEolCalSt2.MCECS_GAINCMDBE;
      |
      | CurrMeasEolAvrgCntr = 0;
      | CurrMeasEolTranCntr = 0;
      |
      | CurrMeasTmpMotCurrAdcVlySum1 = 0;
      | CurrMeasTmpMotCurrAdcVlySum2 = 0;}
  (junction 238) -> (junction 104) [order 1] : [abs(MotCurrAvrgB - MotCurrOffsZeroAvrgB) > ARCHGLBPRM_FLOATZEROTHD_ULS_F32 ...
      | && abs(MotCurrAvrgE - MotCurrOffsZeroAvrgE) > ARCHGLBPRM_FLOATZEROTHD_ULS_F32]
      |
      | {CurrMeasMotCurrEolGainB = CurrMeasEolGainNumer / abs(MotCurrAvrgB - MotCurrOffsZeroAvrgB);
      | CurrMeasMotCurrEolGainE = CurrMeasEolGainNumer / abs(MotCurrAvrgE - MotCurrOffsZeroAvrgE);
      |
      | CurrMeasMotCurrEolCalSt = MotCurrEolCalSt2.MCECS_GAINCMDCF;
      |
      | CurrMeasEolAvrgCntr = 0;
      | CurrMeasEolTranCntr = 0;
      |
      | CurrMeasTmpMotCurrAdcVlySum1 = 0;
      | CurrMeasTmpMotCurrAdcVlySum2 = 0;}
  (junction 241) -> (junction 98) [order 1] : [abs(MotCurrAvrgC - MotCurrOffsZeroAvrgC) > ARCHGLBPRM_FLOATZEROTHD_ULS_F32 ...
      | && abs(MotCurrAvrgF - MotCurrOffsZeroAvrgF) > ARCHGLBPRM_FLOATZEROTHD_ULS_F32]
      |
      | {CurrMeasMotCurrEolGainC = CurrMeasEolGainNumer / abs(MotCurrAvrgC - MotCurrOffsZeroAvrgC);
      | CurrMeasMotCurrEolGainF = CurrMeasEolGainNumer / abs(MotCurrAvrgF - MotCurrOffsZeroAvrgF);
      |
      | CurrMeasMotCurrEolCalSt = MotCurrEolCalSt2.MCECS_CMDSAFEST;
      |
      | CurrMeasEolAvrgCntr = 0;
      | CurrMeasEolTranCntr = 0;
      |
      | CurrMeasTmpMotCurrAdcVlySum1 = 0;
      | CurrMeasTmpMotCurrAdcVlySum2 = 0;}
  (junction 120) -> (junction 297)
  (junction 297) -> (junction 299) [order 2]
  (junction 299) -> (junction 279) : {CurrMeasMotCurrEolCalSt = MotCurrEolCalSt2.MCECS_CMDSAFEST;
      | MotCurrNtcSet = SetNtcSts(EolGainOutOfRng, GainFltParam, 1, 0);
      | CurrMeasEolAvrgCntr = 0;
      | CurrMeasEolTranCntr = 0;
      | EolGainSts = GainFltParam * 4;}
  (junction 297) -> (junction 294) [order 1] : [GainRngChkABC == 1 && GainRngChkDEF == 1]
      | {CurrMeasMotCurrEolCalSt = MotCurrEolCalSt2.MCECS_OFFSCMDSTRT;
      | CurrMeasEolAvrgCntr = 0;
      | CurrMeasEolTranCntr = 0;}
  (junction 294) -> (junction 301) [order 2]
  (junction 301) -> (junction 302) : {MotCurrNtcSet = SetNtcSts(EolGainOutOfRng, 16, 1, 0);
      | EolGainSts = 64;
      | CurrMeasMotCurrEolCalSt = MotCurrEolCalSt2.MCECS_CMDSAFEST;}
  (junction 294) -> (junction 121) [order 1] : [(DiagcStsIvtr1Inactv == 0 || DiagcStsIvtr2Inactv == 0)]
      | {MotCurrNtcSet = SetNtcSts(EolGainOutOfRng, 0, 0, 0);
      | WrNvm();
      | EolGainSts = 2;}
  (junction 110) -> (junction 309)
  (junction 309) -> (junction 91)
  (junction 91) -> (junction 104)
  (junction 104) -> (junction 98)
  (junction 98) -> (junction 278)
  (junction 278) -> (junction 279)
  (junction 279) -> (junction 121)
  (junction 131) -> (junction 121)
  (junction 121) -> (junction 287)
  data: NTCNr function_input; ParamBit function_input; MotCurrNtcSet function_output; NTCSts function_input; NTCDebStep function_input; MotCurrAdcVlyA input; MotCurrAdcVlyB input; MotCurrAdcVlyC input; MotCurrAdcVlyD input; MotCurrAdcVlyE input; MotCurrAdcVlyF input; CurrMeasEolGainNrOfSample input; MotCurrOffsZeroAvrgA input; MotCurrOffsZeroAvrgB input; MotCurrOffsZeroAvrgC input; MotCurrOffsZeroAvrgD input; MotCurrOffsZeroAvrgE input; MotCurrOffsZeroAvrgF input; DiagcStsIvtr1Inactv input; DiagcStsIvtr2Inactv input; ELECGLBPRM_IVTRCNT_CNT_U08 input; CurrMeasMotCurrEolGainA output single; CurrMeasMotCurrEolGainB output single; CurrMeasMotCurrEolGainC output single; CurrMeasMotCurrEolGainD output single; CurrMeasMotCurrEolGainE output single; CurrMeasEolGainMin input; CurrMeasEolGainMax input; CurrMeasMotCurrEolGainF output single; CurrMeasEolGainNumer input; CurrMeasMotCurrEolCalSt output Enum: MotCurrEolCalSt2; MotCurrAvrgA local double; MotCurrAvrgB local double; MotCurrAvrgC local double; MotCurrAvrgD local double; MotCurrAvrgE local double; MotCurrAvrgF local double; MotCurrNtcSet local double; NTC1ED constant double; MotCurrEolGainNTC local single; CurrMeasEolMaxMotVel input; CurrMeasEolTranCntrThd input; MotCurrEolOffsProcFlg input boolean; MotVelMrf input; VehSpd input; VehSpdVld input; CurrMeasMotCurrEolCalStPrev input; EolGainStsPrev input; EolGainSts output uint8; CurrMeasEolAvrgCntrPrev input uint16; CurrMeasEolTranCntrPrev input; CurrMeasEolAvrgCntr output uint16; CurrMeasEolTranCntr output uint8; CurrMeasTmpMotCurrAdcVlySum1Prev input; CurrMeasTmpMotCurrAdcVlySum2Prev input; CurrMeasTmpMotCurrAdcVlySum1 output single; CurrMeasTmpMotCurrAdcVlySum2 output single; EolGainOutOfRng constant double; GainRngChkABC local double; GainRngChkDEF local double; GainFltParam local double; ARCHGLBPRM_FLOATZEROTHD_ULS_F32 parameter
